simulink model "Struct_Bus"  (R2016b)
settings: Solver=FixedStepDiscrete  StartTime=0.0  StopTime=10.0  RelTol=1e-3
settings Model: Creator=3essawy  LastModifiedBy=3essawy
settings OptimizationCC: DefaultParameterBehavior=Inlined
settings DebuggingCC: ParameterTunabilityLossMsg=error
settings RTWCC: SystemTargetFile=ert.tlc  GenCodeOnly=on  TemplateMakefile=ert_default_tmf  Description=Embedded Coder  GenerateReport=on  IncludeHyperlinkInReport=on  LaunchReport=on  GenerateTraceInfo=on  GenerateTraceReport=on  GenerateTraceReportSl=on  GenerateTraceReportSf=on  GenerateTraceReportEml=on
settings CodeAppCC: ForceParamTrailComments=on  IgnoreCustomStorageClasses=off  OperatorAnnotations=on  SimulinkDataObjDesc=on  SFDataObjDesc=on  MATLABFcnDesc=on  InsertBlockDesc=on  MATLABSourceComments=on
settings ERTTargetCC: TargetLangStandard=C99 (ISO)  GenerateSampleERTMain=on  InlinedParameterPlacement=NonHierarchical  ERTCustomFileTemplate=example_file_process.tlc  EnableUserReplacementTypes=on

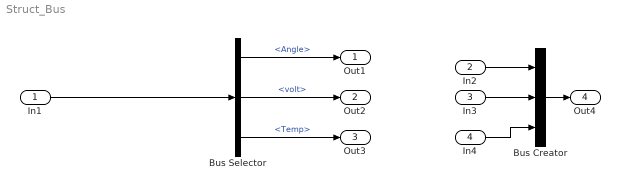
== system Struct_Bus ==
  In1 : Inport  OutDataTypeStr=Bus: Fault_t
  In2 : Inport  Port=2  OutDataTypeStr=uint8
  In3 : Inport  Port=3  OutDataTypeStr=uint8
  In4 : Inport  Port=4  OutDataTypeStr=uint8
  Bus Creator : BusCreator  Inputs=3
  Bus Selector : BusSelector  OutputSignals=Angle,volt,Temp
  Out1 : Outport
  Out2 : Outport  Port=2
  Out3 : Outport  Port=3
  Out4 : Outport  Port=4  OutDataTypeStr=Bus: Fault_t
  wires:
  In1/1 -> Bus Selector/1
  Bus Selector/1 -> Out1/1  "<Angle>"
  Bus Selector/2 -> Out2/1  "<volt>"
  Bus Selector/3 -> Out3/1  "<Temp>"
  In2/1 -> Bus Creator/1
  In3/1 -> Bus Creator/2
  In4/1 -> Bus Creator/3
  Bus Creator/1 -> Out4/1
